simulink model "tvc_lqr_gain_scheduled_extended_states"  (R2025b)
settings: Solver=VariableStepAuto  StartTime=0.0  StopTime=25  RelTol=1e-3
values from neighbouring files (symbols this model uses):
  A_sys = [ 0, 1, 0, 0, 0, 0 ... (first row only)    [starship_tvc_extended_states.m]
  B_sys = [0, 0, 0, 0; K_phi, -K_phi, 0, 0; 0, 0, 0, 0; 0, 0, Ctp_max, 0; 0, 0, 0, 0; 0, 0, 0, Cty_max]    [starship_tvc_extended_states.m]
  C_sys = eye(6)    [starship_tvc_extended_states.m]
  D_sys = zeros(6, 4)    [starship_tvc_extended_states.m]
  flightplan_height = [ascent, descent]    [starship_tvc_extended_states.m]
  g = 9.81    [starship_tvc_extended_states.m]
  Gain_Index = 1:24    [starship_tvc_extended_states.m]
  K_schedule_data = zeros(length(T_schedule), 24)    [starship_tvc_extended_states.m]
  launchtime = 2    [starship_tvc_extended_states.m]
  m = 2.5    [starship_tvc_extended_states.m]
  pitch_demand_conversion = pitch_offset_demand * pi/180    (= 0.0872664625997)    [starship_tvc_extended_states.m]
  roll_demand_conversion = roll_demand * pi/180    (= 0.349065850399)    [starship_tvc_extended_states.m]
  T_max = T_schedule(end)    [starship_tvc_extended_states.m]
  T_schedule = g * [0.11, 0.43, 0.95, 1.5, 1.91, 2.45, 3.1, 3.5, 3.9, 4.23]    [starship_tvc_extended_states.m]
  tau_motor = 50    [starship_tvc_extended_states.m]
  Time_Vector = linspace(launchtime, Total_Simulation_Time, length(flightplan_height))    [starship_tvc_extended_states.m]
  Total_Simulation_Time = 21    [starship_tvc_extended_states.m]
  wind_gust_duration = 2    [starship_tvc_extended_states.m]
libraries: simulink_extras x4, aerolibanim x2, aerolibfltsims x2, slpidlib x1
settings Model: Creator=freak  LastModifiedBy=freak

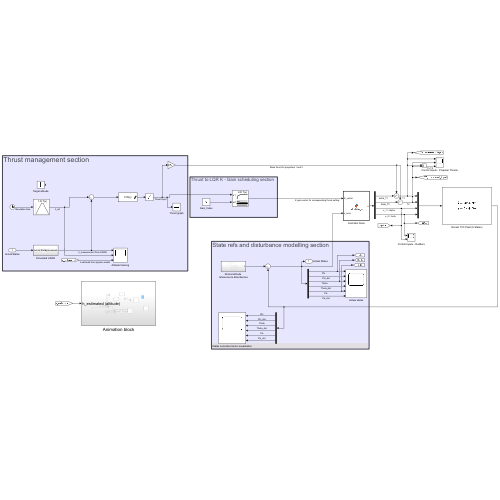
[thumbnail: Simulink's stored preview of the top-level diagram]
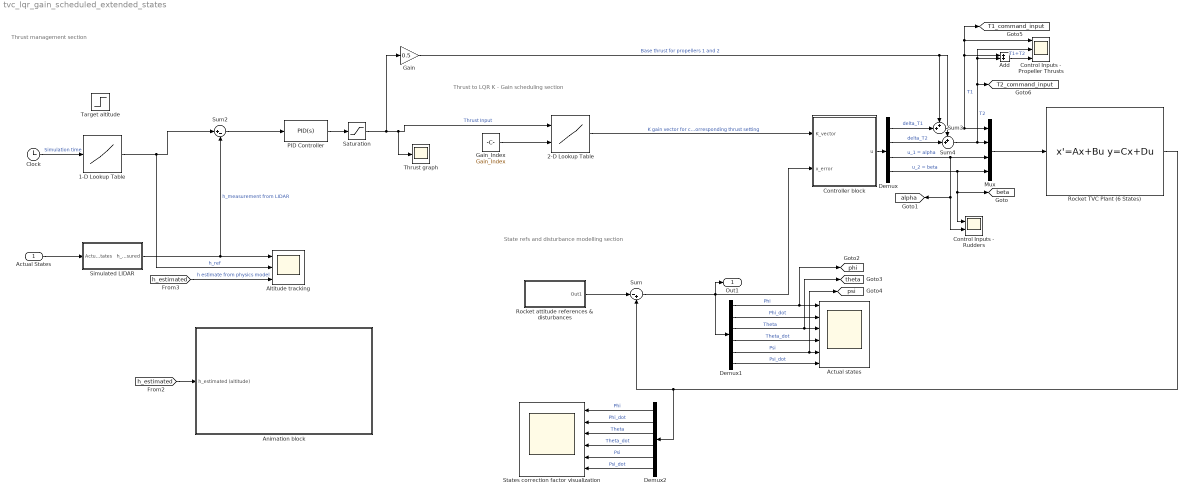
== system tvc_lqr_gain_scheduled_extended_states ==
  note: State refs and disturbance modelling section
  note: Thrust to LQR K - Gain scheduling section
  note: Thrust management section
  Actual States : Inport
  1-D Lookup Table : Lookup_n-D  NumberOfTableDimensions=1  BreakpointsForDimension1=Time_Vector  Table=flightplan_height  ExtrapMethod=Clip  UseLastTableValue=on  InternalRulePriority=Speed  RndMeth=Simplest
  2-D Lookup Table : Lookup_n-D  BreakpointsSpecification=Even spacing  BreakpointsForDimension1=T_schedule  BreakpointsForDimension2=Gain_Index  IndexSearchMethod=Evenly spaced points  Table=K_schedule_data  InternalRulePriority=Speed  RndMeth=Simplest
      settings: InputPortMap=u0,u1
  Actual states : Scope  NumInputPorts=6
      settings: ActiveDisplayYMinimum=-0.7847971904521015  ActiveDisplayYMaximum=0.81222294855788724
  Add : Sum
  Altitude tracking : Scope  NumInputPorts=3
      settings: ActiveDisplayYMinimum=-1.7642569245834547  ActiveDisplayYMaximum=4.7752748155001949  DataLoggingVariableName=ScopeData4
  Animation block : Subsystem
  Clock : Clock
  Control Inputs - Propeller Thrusts : Scope  NumInputPorts=3
      settings: ActiveDisplayYMinimum=-5.1870375  ActiveDisplayYMaximum=46.683337500000007  DataLoggingVariableName=ScopeData6
  Control Inputs - Rudders : Scope  NumInputPorts=2
      settings: ActiveDisplayYMinimum=-2.9579809113570303  ActiveDisplayYMaximum=2.9231355464726687
  Controller block : MATLAB Function  TreatAsAtomicUnit=on
  Demux : Demux
  Demux1 : Demux  Outputs=6
  Demux2 : Demux  Outputs=6
  Gain : Gain  Gain=0.5
  Gain_Index : Constant  Value=Gain_Index
  Mux : Mux
  PID Controller : slpidlib/PID Controller  Controller=PID  Form=Parallel  TimeDomain=Continuous-time  UseExternalTs=off  SampleTime=-1  IntegratorMethod=Forward Euler  FilterMethod=Forward Euler  ControllerParametersSource=internal  P=10  I=20  UseKiTs=off  D=10  UseExternalDerivativeSource=off  N=7  UseFilter=on  TunerSelectOption=Transfer Function Based (PID Tuner App)  InitialConditionSource=internal  InitialConditionForIntegrator=0  InitialConditionForFilter=0  DifferentiatorICPrevScaledInput=0  ExternalReset=none  TrackingMode=off  Kt=1  LimitOutput=on  SatLimitsSource=internal  UpperSaturationLimit=70  LowerSaturationLimit=0  LinearizeAsGain=on  AntiWindupMode=none  Kb=1  LimitIntegrator=off  UpperIntegratorSaturationLimit=inf  LowerIntegratorSaturationLimit=-inf  POutMin=[]  POutMax=[]  IOutMin=[]  IOutMax=[]  DOutMin=[]  DOutMax=[]  NOutMin=[]  NOutMax=[]  SumOutMin=[]  SumOutMax=[]  SaturationOutMin=[]  SaturationOutMax=[]  PParamMin=[]  PParamMax=[]  IParamMin=[]  IParamMax=[]  DParamMin=[]  DParamMax=[]  NParamMin=[]  NParamMax=[]  KbParamMin=[]  KbParamMax=[]  KtParamMin=[]  KtParamMax=[]  KbOutMin=[]  KbOutMax=[]  KtOutMin=[]  KtOutMax=[]  IntegratorOutMin=[]  IntegratorOutMax=[]  FilterOutMin=[]  FilterOutMax=[]  SumI1OutMin=[]  SumI1OutMax=[]  SumI2OutMin=[]  SumI2OutMax=[]  SumI3OutMin=[]  SumI3OutMax=[]  SumI4OutMin=[]  SumI4OutMax=[]  SumDOutMin=[]  SumDOutMax=[]  DifferentiatorOutMin=[]  DifferentiatorOutMax=[]  FilterDiffOutCoefMin=[]  FilterDiffOutCoefMax=[]  ReciprocalOutMin=[]  ReciprocalOutMax=[]  SumDenOutMin=[]  SumDenOutMax=[]  SumNumOutMin=[]  SumNumOutMax=[]  DivideOutMin=[]  DivideOutMax=[]  UdiffTsProdOutMin=[]  UdiffTsProdOutMax=[]  NTsProdOutMin=[]  NTsProdOutMax=[]  UintegralTsProdOutMin=[]  UintegralTsProdOutMax=[]  UngainTsProdOutMin=[]  UngainTsProdOutMax=[]  ClampingZeroOutDataTypeStr=Inherit: Inherit via back propagation  ClampingZeroOutMin=[]  ClampingZeroOutMax=[]  FilterDenConstantOutDataTypeStr=Inherit: Inherit via back propagation  FilterDenConstantOutMin=[]  FilterDenConstantOutMax=[]  PCopyOutDataTypeStr=Inherit: Inherit via back propagation  PCopyOutMin=[]  PCopyOutMax=[]  NCopyOutDataTypeStr=Inherit: Inherit via back propagation  NCopyOutMin=[]  NCopyOutMax=[]  IntegratorContinuousStateAttributes=''  IntegratorStateMustResolveToSignalObject=off  IntegratorRTWStateStorageClass=Auto  FilterContinuousStateAttributes=''  FilterStateMustResolveToSignalObject=off  FilterRTWStateStorageClass=Auto  ParallelPVariant=InternalParameters  IdealPVariant=Disabled  IVariant=InternalParameters  DVariant=InternalParameters  IntegratorVariant=Continuous  SatVariant=Enabled  AWVariant=Passthrough  PCopyVariant=Disabled  TRVariant=Disabled  FdbkBlocksVariant=Forward  IdealPFdbkVariant=Disabled  SatFdbkVariant=Disabled  DerivativeFilterVariant=ContFilter  NVariant=InternalParameters  NCopyVariant=Disabled  FilterICVariant=InternalICsFilter  IntegratorICVariant=InternalICs  ExternalResetVariant=Disabled  TRSumVariant=Passthrough  SumFdbkVariant=Disabled  SumVariant=Sum_PID  TsampFilterVariant=InternalTs  TsampNgainVariant=Passthrough  TsampIntegralVariant=Disabled_SignalSpec  ExternalSaturationOutDataTypeStr=Inherit: Same as second input  DerivativeSourceVariant=ErrorSignal  PreIntVariant=InternalPreInt
  Rocket TVC Plant (6 States) : StateSpace  A=A_sys  B=B_sys  C=C_sys  D=D_sys  InitialCondition=0  ContinuousStateAttributes={'phi', 'phi_dot', 'theta','theta_dot','psi','psi_dot'}
  Rocket attitude references & disturbances : Subsystem
  Saturation : Saturate  UpperLimit=T_max  LowerLimit=0
  Simulated LIDAR : Subsystem
  States correction factor visualization : Scope  NumInputPorts=6
      settings: ActiveDisplayYMinimum=-0.46880516298147618  ActiveDisplayYMaximum=0.45896834599975539  DataLoggingVariableName=ScopeData2
  Sum : Sum  Inputs=|-+
  Sum2 : Sum  Inputs=|+-
  Sum3 : Sum  Inputs=++|
  Sum4 : Sum  Inputs=++|
  Target altitude : Step  Time=launchtime  After=5  SampleTime=0
  Thrust graph : Scope
      settings: ActiveDisplayYMinimum=-1  ActiveDisplayYMaximum=1  DataLoggingVariableName=ScopeData5
  Out1 : Outport  SignalName=Actual States
  tag scope: T1_command_input=global, T2_command_input=global, alpha=global, beta=global, phi=global, psi=global, theta=global
  wires:
  Gain_Index/1 -> 2-D Lookup Table/2
  Controller block/1(u) -> Demux/1
  Sum/1 -> Out1/1, Controller block/2(x_error), Demux1/1
  Mux/1 -> Rocket TVC Plant (6 States)/1
  Demux/4 -> Control Inputs - Rudders/1, [beta], Mux/4  "u_2 = beta"
  Demux/3 -> Control Inputs - Rudders/2, [alpha], Mux/3  "u_1 = alpha"
  2-D Lookup Table/1 -> Controller block/1(K_vector)  "K gain vector for corresponding thrust setting"
  Sum2/1 -> PID Controller/1
  PID Controller/1 -> Saturation/1
  Saturation/1 -> 2-D Lookup Table/1, Thrust graph/1, Gain/1  "Thrust Input"
  Demux/2 -> Sum4/2  "delta_T2"
  Sum4/1 -> [T2_command_input], Add/2, Control Inputs - Propeller Thrusts/2, Mux/2  "T2"
  Gain/1 -> Sum4/1, Sum3/1  "Base thrust for propellers 1 and 2"
  Demux/1 -> Sum3/2  "delta_T1"
  Sum3/1 -> Add/1, [T1_command_input], Control Inputs - Propeller Thrusts/1, Mux/1  "T1"
  [h_estimated] -> Animation block/1(h_estimated (altitude))
  [h_estimated] -> Altitude tracking/3  "h estimate from physics model"
  Simulated LIDAR/1(h_measured) -> Altitude tracking/1, Sum2/2  "h_measurement from LIDAR"
  Actual States/1 -> Simulated LIDAR/1(Actual States)
  Clock/1 -> 1-D Lookup Table/1  "Simulation time"
  1-D Lookup Table/1 -> Altitude tracking/2, Sum2/1  "h_ref"
  Rocket attitude references & disturbances/1(Out1) -> Sum/1
  Add/1 -> Control Inputs - Propeller Thrusts/3  "T1+T2"
  Demux1/5 -> [psi], Actual states/5  "Psi"
  Demux1/4 -> Actual states/4  "Theta_dot"
  Demux1/1 -> [phi], Actual states/1  "Phi"
  Demux1/2 -> Actual states/2  "Phi_dot"
  Demux1/6 -> Actual states/6  "Psi_dot"
  Demux1/3 -> [theta], Actual states/3  "Theta"
  Demux2/5 -> States correction factor visualization/5  "Psi"
  Demux2/4 -> States correction factor visualization/4  "Theta_dot"
  Demux2/1 -> States correction factor visualization/1  "Phi"
  Demux2/2 -> States correction factor visualization/2  "Phi_dot"
  Demux2/6 -> States correction factor visualization/6  "Psi_dot"
  Demux2/3 -> States correction factor visualization/3  "Theta"
  Rocket TVC Plant (6 States)/1 -> Sum/2, Demux2/1

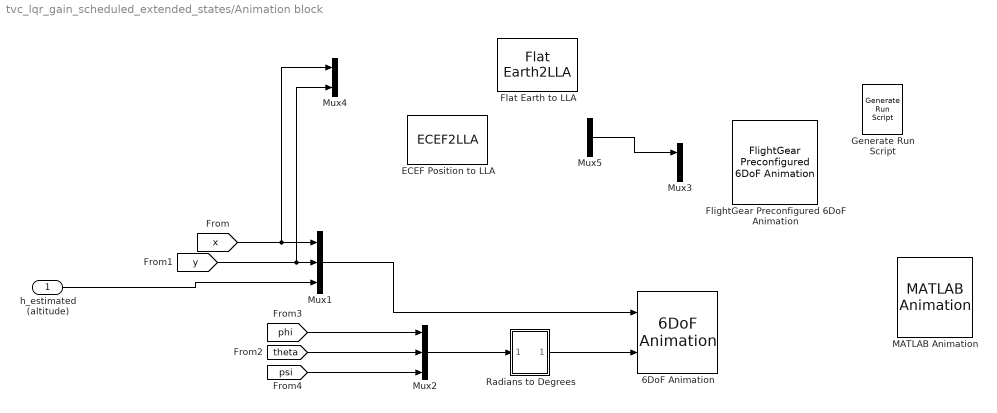
== system tvc_lqr_gain_scheduled_extended_states/Animation block ==
  h_estimated (altitude) : Inport
  6DoF Animation : aerolibanim/6DoF Animation  u1=[-20 80 -20 80 -20 80]  u2=0.1  u3=2  u4=[-5 -5 -5]  u5=Fly alongside  u6=[2 2 1]  u7=90  u8=off
  ECEF Position to LLA : ECEF2LLA
  Flat Earth to LLA : FlatEarth2LLA  psi=90
  FlightGear Preconfigured 6DoF Animation : aerolibfltsims/FlightGear Preconfigured 6DoF Animation  xFlightGearVersion=v2019.1  DestinationIpAddress=127.0.0.1  DestinationPort=5502  SampleTime=1/30  packetVersion=24
  Generate Run Script : aerolibfltsims/Generate Run Script  Architecture=Win64  dataFlow=Send  GeometryModelName=f16  AirportId=KSFO  RunwayId=10L  InitialAltitude=7224  InitialHeading=113  OffsetDistance=4.72  OffsetAzimuth=0  InstallScenery=off  DisableShaders=off  OriginAddress=127.0.0.1  DestinationPort=5502  OriginPort=5505  LocalAddress=127.0.0.1  OutputFileName=launch_rocket.bat  FlightGearBaseDirectory=C:\Program Files\FlightGear 2024.1
  MATLAB Animation : aerolibanim/MATLAB Animation  Tag=Matlab Animation 6 DOF  Vehicles=1  Geometries='astredwedge.mat'  BoundingBoxCoordinates=[-50,50,-50,50,-50,50]  CameraOffset=[-150,-50,0]  CameraViewAngle=2  SampleTime=20  FigurePosition=[1,49,1536,766]
  Mux1 : Mux  Inputs=3
  Mux2 : Mux  Inputs=3
  Mux3 : Mux  Inputs=2
  Mux4 : Mux  Inputs=2
  Mux5 : Mux  Inputs=2
  Radians to Degrees : Subsystem
  wires:
  Mux1/1 -> 6DoF Animation/1
  Radians to Degrees/1(Out1) -> 6DoF Animation/2
  [x] -> Mux4/1, Mux1/1
  [theta] -> Mux2/2
  Mux2/1 -> Radians to Degrees/1(In1)
  [y] -> Mux4/2, Mux1/2
  [phi] -> Mux2/1
  Mux5/1 -> Mux3/1
  [psi] -> Mux2/3
  h_estimated (altitude)/1 -> Mux1/3

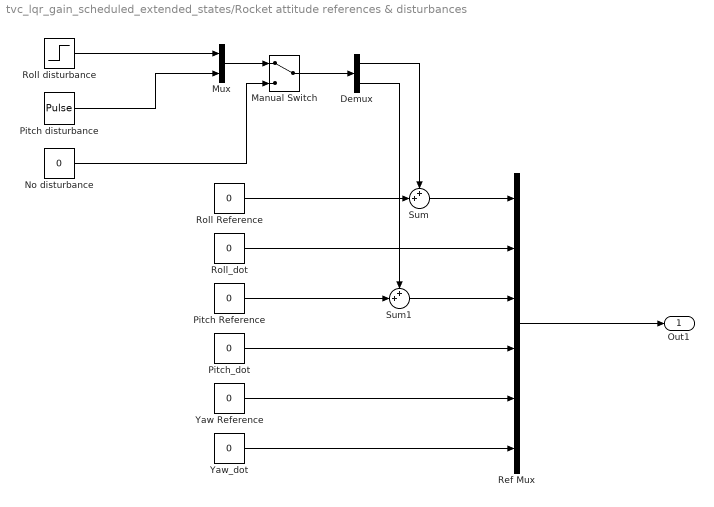
== system tvc_lqr_gain_scheduled_extended_states/Rocket attitude references & disturbances ==
  Demux : Demux  Outputs=2
  Manual Switch : ManualSwitch
  Mux : Mux  Inputs=2
  No disturbance : Constant  Value=0
  Pitch Reference : Constant  Value=0
  Pitch disturbance : DiscretePulseGenerator  PulseType=Time based  Amplitude=pitch_demand_conversion  Period=Total_Simulation_Time  PulseWidth=(wind_gust_duration/Total_Simulation_Time)*100  PhaseDelay=4 + launchtime
  Pitch_dot : Constant  Value=0
  Ref Mux : Mux  Inputs=6
  Roll Reference : Constant  Value=0
  Roll disturbance : Step  Time=13 + launchtime  After=roll_demand_conversion  SampleTime=0
  Roll_dot : Constant  Value=0
  Sum : Sum  Inputs=++|
  Sum1 : Sum  Inputs=++|
  Yaw Reference : Constant  Value=0
  Yaw_dot : Constant  Value=0
  Out1 : Outport
  wires:
  Roll_dot/1 -> Ref Mux/2
  Yaw Reference/1 -> Ref Mux/5
  Pitch_dot/1 -> Ref Mux/4
  Yaw_dot/1 -> Ref Mux/6
  Ref Mux/1 -> Out1/1
  Manual Switch/1 -> Demux/1
  Demux/2 -> Sum1/1
  Sum1/1 -> Ref Mux/3
  Pitch Reference/1 -> Sum1/2
  Sum/1 -> Ref Mux/1
  Demux/1 -> Sum/1
  Roll Reference/1 -> Sum/2
  Mux/1 -> Manual Switch/1
  Pitch disturbance/1 -> Mux/2
  Roll disturbance/1 -> Mux/1
  No disturbance/1 -> Manual Switch/2

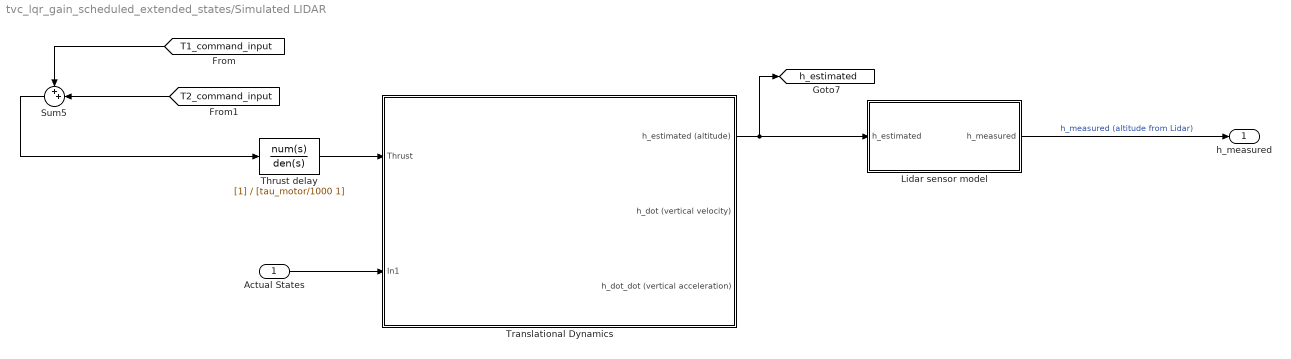
== system tvc_lqr_gain_scheduled_extended_states/Simulated LIDAR ==
  Actual States : Inport
  Lidar sensor model : Subsystem
  Sum5 : Sum  Inputs=++|
  Thrust delay : TransferFcn  Denominator=[tau_motor/1000 1]
  Translational Dynamics : Subsystem
  h_measured : Outport
  tag scope: h_estimated=global
  wires:
  [T2_command_input] -> Sum5/2
  Actual States/1 -> Translational Dynamics/2(In1)
  [T1_command_input] -> Sum5/1
  Thrust delay/1 -> Translational Dynamics/1(Thrust)
  Sum5/1 -> Thrust delay/1
  Translational Dynamics/1(h_estimated (altitude)) -> [h_estimated], Lidar sensor model/1(h_estimated)
  Lidar sensor model/1(h_measured) -> h_measured/1  "h_measured (altitude from Lidar)"

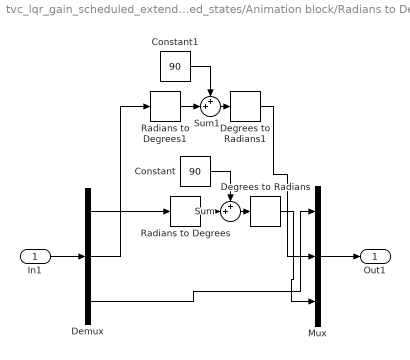
== system tvc_lqr_gain_scheduled_extended_states/Animation block/Radians to Degrees ==
  In1 : Inport
  Constant : Constant  Value=90
  Constant1 : Constant  Value=90
  Degrees to Radians : simulink_extras/Transformations/Degrees to Radians
  Degrees to Radians1 : simulink_extras/Transformations/Degrees to Radians
  Demux : Demux  Outputs=3
  Mux : Mux  Inputs=3
  Radians to Degrees : simulink_extras/Transformations/Radians to Degrees
  Radians to Degrees1 : simulink_extras/Transformations/Radians to Degrees
  Sum : Sum  Inputs=++|
  Sum1 : Sum  Inputs=++|
  Out1 : Outport
  wires:
  Demux/1 -> Radians to Degrees/1
  Radians to Degrees/1 -> Sum/2
  Constant/1 -> Sum/1
  Sum/1 -> Degrees to Radians/1
  In1/1 -> Demux/1
  Mux/1 -> Out1/1
  Degrees to Radians/1 -> Mux/3
  Demux/3 -> Mux/1
  Degrees to Radians1/1 -> Mux/2
  Sum1/1 -> Degrees to Radians1/1
  Demux/2 -> Radians to Degrees1/1
  Radians to Degrees1/1 -> Sum1/2
  Constant1/1 -> Sum1/1

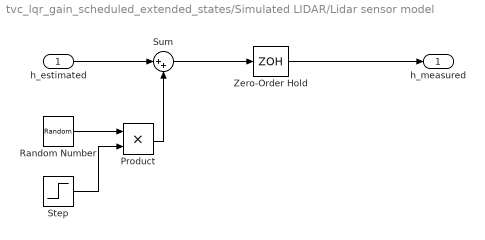
== system tvc_lqr_gain_scheduled_extended_states/Simulated LIDAR/Lidar sensor model ==
  h_estimated : Inport
  Product : Product
  Random Number : RandomNumber  Variance=0.001  SampleTime=0.1
  Step : Step  Time=launchtime  SampleTime=0
  Sum : Sum  Inputs=|++
  Zero-Order Hold : ZeroOrderHold  SampleTime=0.01
  h_measured : Outport
  wires:
  h_estimated/1 -> Sum/1
  Sum/1 -> Zero-Order Hold/1
  Zero-Order Hold/1 -> h_measured/1
  Product/1 -> Sum/2
  Random Number/1 -> Product/1
  Step/1 -> Product/2

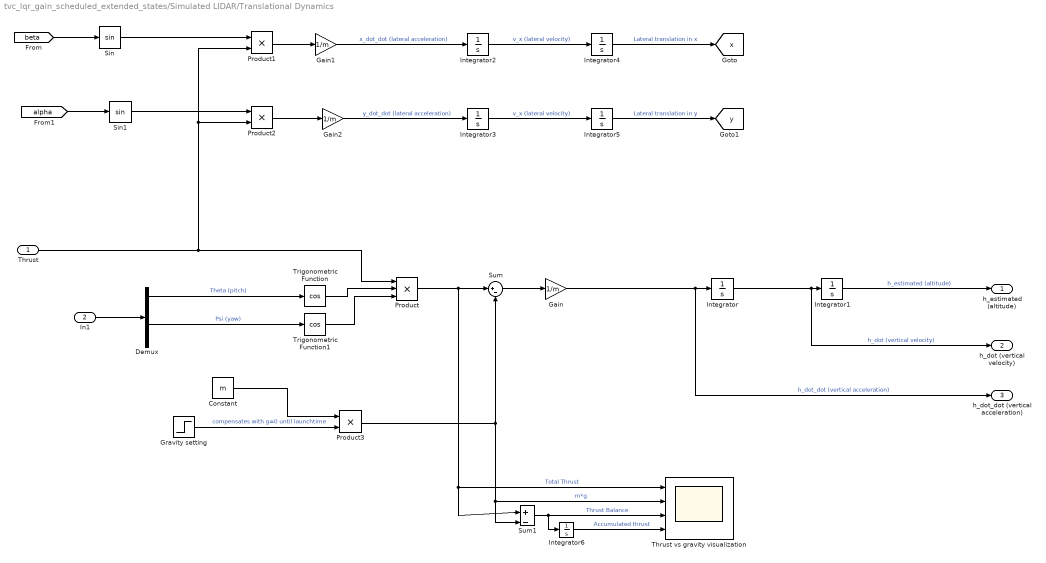
== system tvc_lqr_gain_scheduled_extended_states/Simulated LIDAR/Translational Dynamics ==
  Thrust : Inport
  In1 : Inport  Port=2
  Constant : Constant  Value=m
  Demux : Demux
  Gain : Gain  Gain=1/m
  Gain1 : Gain  Gain=1/m
  Gain2 : Gain  Gain=1/m
  Gravity setting : Step  Time=launchtime  After=g  SampleTime=0
  Integrator{,1..6} (7 alike) : Integrator
  Product : Product  Inputs=3
  Product1 : Product
  Product2 : Product
  Product3 : Product
  Sin : Trigonometry
  Sin1 : Trigonometry
  Sum : Sum  Inputs=|+-
  Sum1 : Sum  Inputs=|+-
  Thrust vs gravity visualization : Scope  NumInputPorts=4
      settings: ActiveDisplayYMinimum=-32.650495240787542  ActiveDisplayYMaximum=48.604457167087851  DataLoggingVariableName=ScopeData3
  Trigonometric Function : Trigonometry  Operator=cos
  Trigonometric Function1 : Trigonometry  Operator=cos
  h_estimated (altitude) : Outport
  h_dot (vertical velocity) : Outport  Port=2
  h_dot_dot (vertical acceleration) : Outport  Port=3
  tag scope: x=global, y=global
  wires:
  Demux/3 -> Trigonometric Function1/1  "Psi (yaw)"
  Trigonometric Function1/1 -> Product/3
  Trigonometric Function/1 -> Product/2
  Thrust/1 -> Product2/2, Product1/2, Product/1
  Product/1 -> Sum1/1, Thrust vs gravity visualization/1, Sum/1  "Total Thrust"
  Sum/1 -> Gain/1
  Gain/1 -> h_dot_dot (vertical acceleration)/1, Integrator/1  "h_dot_dot (vertical acceleration)"
  Integrator/1 -> h_dot (vertical velocity)/1, Integrator1/1  "h_dot (vertical velocity)"
  Integrator1/1 -> h_estimated (altitude)/1  "h_estimated (altitude)"
  In1/1 -> Demux/1
  Demux/1 -> Trigonometric Function/1  "Theta (pitch)"
  [beta] -> Sin/1
  [alpha] -> Sin1/1
  Sin/1 -> Product1/1
  Sin1/1 -> Product2/1
  Product1/1 -> Gain1/1
  Product2/1 -> Gain2/1
  Gain1/1 -> Integrator2/1  "x_dot_dot (lateral acceleration)"
  Gain2/1 -> Integrator3/1  "y_dot_dot (lateral acceleration)"
  Integrator2/1 -> Integrator4/1  "v_x (lateral velocity)"
  Integrator3/1 -> Integrator5/1  "v_x (lateral velocity)"
  Integrator4/1 -> [x]  "Lateral translation in x"
  Integrator5/1 -> [y]  "Lateral translation in y"
  Gravity setting/1 -> Product3/2  "compensates with g=0 until launchtime"
  Product3/1 -> Sum/2, Sum1/2, Thrust vs gravity visualization/2  "m*g"
  Constant/1 -> Product3/1
  Sum1/1 -> Integrator6/1, Thrust vs gravity visualization/3  "Thrust Balance"
  Integrator6/1 -> Thrust vs gravity visualization/4  "Accumulated thrust"

== matlab function tvc_lqr_gain_scheduled_extended_states/Controller block ==
  data: K_vector input; u output; x_error input
function u = calculate_u(K_vector, x_error)
% u = -K * x_error; 
% Inputs:
%   K_vector: 24x1 or 1x24 vector of gains from Lookup Table (4x6 matrix)
%   x_error: 6x1 State error vector [phi_err; d_phi_err; theta_err; d_theta_err; psi_err; d_psi_err]

% Reshape vector back into 4x6 Gain Matrix that is equal to K_curr
K = reshape(K_vector, 4, 6)
% K = K_vector;

% Calculate Control Deviations
u = -K * x_error;

% Output u is the 4x1 control input: u = [delta_T1; delta_T2; alpha; beta]
end
